simulink model "Robustofinal"  (R2021b)
settings: Solver=VariableStepAuto  StartTime=0.0  StopTime=3  FixedStep=0.000001  RelTol=1e-3
values from neighbouring files (symbols this model uses):
  C = 2500*10^-6    (= 0.0025)    [parametrosRs.m]
  Em = 80    [parametrosRs.m]
  epsilon = 0.1    [parametrosRs.m]
  k1 = 103    [parametrosRs.m]
  k2 = 1000    [parametrosRs.m]
  k3 = 3000    [parametrosRs.m]
  L = 10*10^-3    (= 0.01)    [parametrosRs.m]
  R = 0.1    [parametrosRs.m]
  Rl = 33.33    [parametrosRs.m]
  w = 60    [parametrosRs.m]
  x2d = 0    [parametrosRs.m]
  x3d = 48    [parametrosRs.m]
libraries: spsIGBTDiodeLib x6, eeTransforms x5, spsCurrentMeasurementLib x4, spsSeriesRLCBranchLib x4, spsVoltageMeasurementLib x4, spsACVoltageSourceLib x3, simulink x1, spsDCVoltageSourceLib x1, spsGroundLib x1, spsSVPWMGenerator2LevelLib x1, spsVariableResistorLib x1, spspowerguiLib x1
settings Model: Creator=CIO  LastModifiedBy=LAPONE

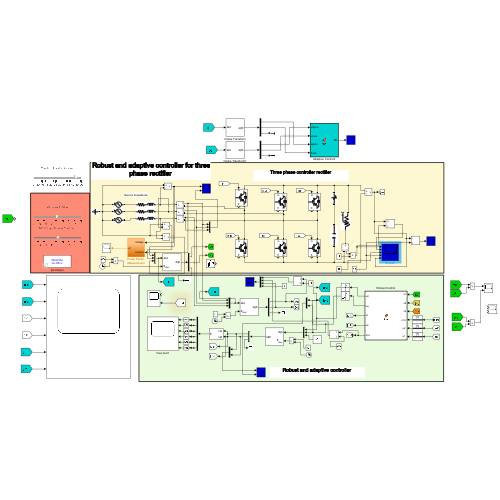
[thumbnail: Simulink's stored preview of the top-level diagram]
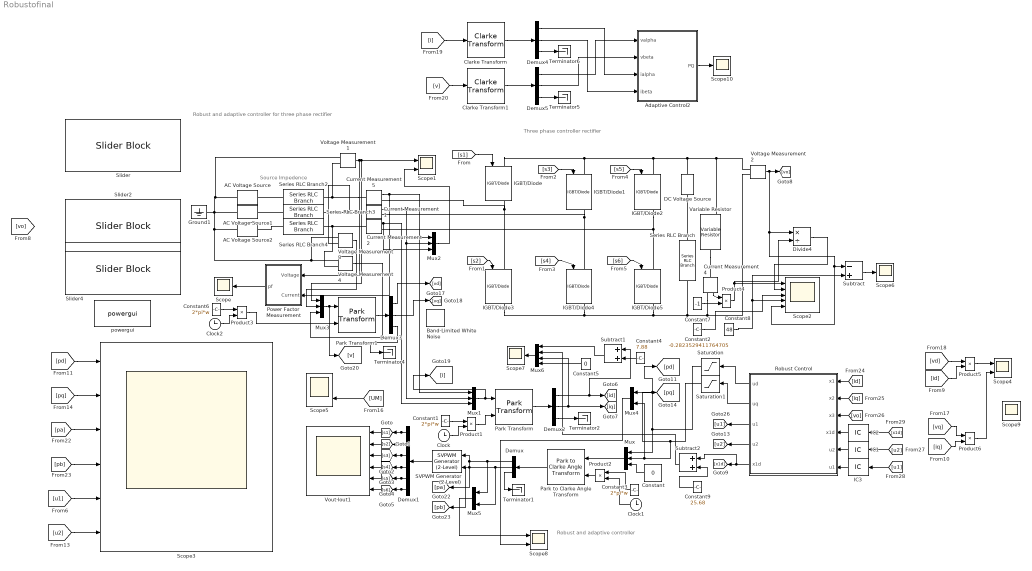
== system Robustofinal ==
  note: Source Impedence
  note: Three phase controller rectifier
  note: Robust and adaptive controller
  note: Robust and adaptive controller for three phase rectifier
  AC Voltage Source : spsACVoltageSourceLib/AC Voltage Source  Amplitude=Em  Phase=0  Frequency=w  SampleTime=0  Measurements=None  BusType=swing  Pref=10e3  Qref=0  Qmin=-inf  Qmax=+inf
  AC Voltage Source1 : spsACVoltageSourceLib/AC Voltage Source  Amplitude=Em  Phase=240  Frequency=w  SampleTime=0  Measurements=None  BusType=swing  Pref=10e3  Qref=0  Qmin=-inf  Qmax=+inf
  AC Voltage Source2 : spsACVoltageSourceLib/AC Voltage Source  Amplitude=Em  Phase=120  Frequency=w  SampleTime=0  Measurements=None  BusType=swing  Pref=10e3  Qref=0  Qmin=-inf  Qmax=+inf
  Adaptive Control2 : MATLAB Function  TreatAsAtomicUnit=on
  Band-Limited White Noise : simulink/Sources/Band-Limited White Noise  Cov=[0.001]  Ts=0.001  seed=[23341]
  Clarke Transform : eeTransforms/Clarke Transform  PowerInvariant=off
      settings: SourceProductBaseCode=PS
  Clarke Transform1 : eeTransforms/Clarke Transform  PowerInvariant=off
      settings: SourceProductBaseCode=PS
  Clock : Clock
  Clock1 : Clock
  Clock2 : Clock
  Constant : Constant  Value=0
  Constant1 : Constant  Value=2*pi*w
  Constant2 : Constant  Value=-0.2823529411764705
  Constant3 : Constant  Value=2*pi*w
  Constant4 : Constant  Value=7.88
  Constant5 : Constant  Value=0
  Constant6 : Constant  Value=2*pi*w
  Constant7 : Constant  Value=-1
  Constant8 : Constant  Value=48
  Constant9 : Constant  Value=25.68
  Current Measurement{1..2,4..5} (4 alike) : spsCurrentMeasurementLib/Current Measurement  PhasorSimulation=off  OutputType=Magnitude  PSBequivalent=0
  DC Voltage Source : spsDCVoltageSourceLib/DC Voltage Source  Amplitude=0.0941176470588232  Measurements=None
  Demux{,2..5} (5 alike) : Demux  Outputs=3
  Demux1 : Demux  Outputs=6
  Divide4 : Product  Inputs=*/
  Ground1 : spsGroundLib/Ground  LConnTagsString=a
  IC1 : InitialCondition
  IC2 : InitialCondition
  IC3 : InitialCondition
  IGBT/Diode{,1..5} (6 alike) : spsIGBTDiodeLib/IGBT//Diode  Ron=1e-3  Rs=1e5  Cs=inf  Measurements=on
  Mux{,1..3} (4 alike) : Mux  Inputs=3
  Mux4 : Mux  Inputs=2
  Mux5 : Mux  Inputs=2
  Mux6 : Mux
  Park Transform : eeTransforms/Park Transform  AxisAlignment=D-axis  PowerInvariant=off
  Park Transform1 : eeTransforms/Park Transform  AxisAlignment=D-axis  PowerInvariant=off
  Park to Clarke Angle Transform : eeTransforms/Park to Clarke Angle Transform  AxisAlignment=D-axis
      settings: SourceProductBaseCode=PS
  Power Factor Measurement : Subsystem
  Product{1..6} (6 alike) : Product
  Robust Control : MATLAB Function  TreatAsAtomicUnit=on
  SVPWM Generator (2-Level) : spsSVPWMGenerator2LevelLib/SVPWM Generator (2-Level)  InputType=alpha-beta components  SwitchingPattern=Pattern #1  Fc=10000  ParUref=[0.8 -30 50]  Ts=0
      settings: SourceProductBaseCode=PS
  Saturation : Saturate  UpperLimit=50  LowerLimit=-50
  Saturation1 : Saturate  UpperLimit=25  LowerLimit=-25
  Scope{,6..7,10} (4 alike) : Scope
  Scope{1,4..5,8..9} (5 alike) : Scope  NumInputPorts=2
  Scope2 : Scope  NumInputPorts=5
  Scope3 : Scope  NumInputPorts=6
  Series RLC Branch : spsSeriesRLCBranchLib/Series RLC Branch  LConnTagsString=__new0  RConnTagsString=__new0  BranchType=C  Resistance=5  Inductance=1e-3  SetiL0=off  InitialCurrent=0  Capacitance=C  Setx0=off  InitialVoltage=0  Measurements=None
  Series RLC Branch2 : spsSeriesRLCBranchLib/Series RLC Branch  LConnTagsString=__new0  RConnTagsString=__new0  BranchType=RL  Resistance=R  Inductance=L  SetiL0=off  InitialCurrent=0  Capacitance=200e-6  Setx0=off  InitialVoltage=0  Measurements=Branch voltage and current
  Series RLC Branch3 : spsSeriesRLCBranchLib/Series RLC Branch  LConnTagsString=__new0  RConnTagsString=__new0  BranchType=RL  Resistance=R  Inductance=L  SetiL0=off  InitialCurrent=0  Capacitance=200e-6  Setx0=off  InitialVoltage=0  Measurements=Branch voltage and current
  Series RLC Branch4 : spsSeriesRLCBranchLib/Series RLC Branch  LConnTagsString=__new0  RConnTagsString=__new0  BranchType=RL  Resistance=R  Inductance=L  SetiL0=off  InitialCurrent=0  Capacitance=200e-6  Setx0=off  InitialVoltage=0  Measurements=Branch voltage and current
  Slider : SliderBlock  ScaleMin=6  ScaleMax=50
  Slider2 : SliderBlock  ScaleMin=-8  ScaleMax=8
  Slider4 : SliderBlock  ScaleMin=-8  ScaleMax=8
  Subtract : Sum  Inputs=-+
  Subtract1 : Sum
  Subtract2 : Sum
  Terminator{1..2,4..6} (5 alike) : Terminator
  Variable Resistor : spsVariableResistorLib/Variable Resistor  Rabsmin=44.92307692307692
      settings: SourceProductBaseCode=PS
  Voltage Measurement{1..4} (4 alike) : spsVoltageMeasurementLib/Voltage Measurement  PhasorSimulation=off  OutputType=Magnitude  PSBequivalent=0
  Vout-Iout1 : Scope  NumInputPorts=6
  powergui : spspowerguiLib/powergui  Priority=1  SimulationMode=Discrete  SampleTime=1e-6  frequency=60  Iterations=50  frequencyindice=0  Pbase=100e6  ErrMax=1e-4  UnitsV=kV  UnitsW=MW  buscounter=0  FunctionMessages=off  echomessages=off  EnableUseOfTLC=off  CurrentSourceSwitches=off  DisableSnubberDevices=off  DisableRonSwitches=off  DisableVfSwitches=off  DisplayEquations=off  AutomaticDiscreteSolvers=off  SolverType=Tustin/Backward Euler (TBE)  Interpol=off  ExternalGateDelay=off  methode=off  Ts=0  x0status=blocks  SPID=off  SwTol=0  HookPort=off  NonlinearTolerance=0  nMaxIteration=15  ContinueOnMaxIteration=off  RestoreLinks=warning  ResistiveCurrentMeasurement=off  Frange=[0:2:500]  Ylog=off  Xlog=on  ShowGrid=off  save=off  variable=ZData  structure=0  ZoomFFT=on  StartTime=0.0  cycles=1  DisplayStyle=1  fundamental=60  FreqAxis=off  MaxFrequency=1000  frequencyindicesteady=1  RmsSteady=1  display=off
  wires:
  Constant4/1 -> Subtract1/2
  Park to Clarke Angle Transform/1 -> Demux/1
  Clock1/1 -> Product2/2
  Product2/1 -> Park to Clarke Angle Transform/2
  Clock/1 -> Product1/2
  Demux2/3 -> Terminator2/1
  Divide4/1 -> Scope2/2
  Product1/1 -> Park Transform/2
  Constant8/1 -> Subtract/2, Scope2/4
  Constant1/1 -> Product1/1
  Current Measurement2/1 -> Mux2/3, Mux1/3
  Constant3/1 -> Product2/1
  [s2] -> IGBT/Diode3/1
  Product4/1 -> Divide4/2, Scope2/1
  Current Measurement5/1 -> Power Factor Measurement/2(Current), Mux2/1, Mux1/1
  Mux4/1 -> Scope8/2
  [s3] -> IGBT/Diode1/1
  Demux1/1 -> Vout-Iout1/1, [s1]
  Mux1/1 -> [i], Park Transform/1
  Demux1/5 -> Vout-Iout1/5, [s5]
  Voltage Measurement1/1 -> Power Factor Measurement/1(Voltage), Scope1/1, Mux3/1
  Current Measurement1/1 -> Mux2/2, Mux1/2
  Constant/1 -> Mux/3
  Saturation/1 -> Mux4/1, [pd], Mux/1
  Subtract/1 -> Scope6/1
  Current Measurement4/1 -> Product4/1
  Mux2/1 -> Scope1/2
  SVPWM Generator (2-Level)/1 -> Demux1/1
  Demux/1 -> Mux5/1, SVPWM Generator (2-Level)/1, [pa]
  [s1] -> IGBT/Diode/1
  Demux2/2 -> Mux6/3, [iq]
  Constant2/1 -> Scope2/3
  [s6] -> IGBT/Diode5/1
  Demux1/2 -> Vout-Iout1/2, [s2]
  [s4] -> IGBT/Diode4/1
  Park Transform/1 -> Demux2/1
  Voltage Measurement2/1 -> Divide4/1, Scope2/5, Subtract/1, [vo]
  Mux/1 -> Park to Clarke Angle Transform/1
  Mux6/1 -> Scope7/1
  Demux1/4 -> Vout-Iout1/4, [s4]
  Demux/2 -> Mux5/2, [pb], SVPWM Generator (2-Level)/2
  Demux1/3 -> Vout-Iout1/3, [s3]
  [s5] -> IGBT/Diode2/1
  Demux1/6 -> Vout-Iout1/6, [s6]
  Saturation1/1 -> [pq], Mux4/2, Mux/2
  Demux/3 -> Terminator1/1
  Mux5/1 -> Scope8/1
  Constant7/1 -> Product4/2
  Power Factor Measurement/1(pf) -> Scope/1
  [UM] -> Scope5/2
  Constant5/1 -> Mux6/4
  Demux2/1 -> Subtract1/1, [id]
  Mux3/1 -> [v], Park Transform1/1
  Park Transform1/1 -> Demux3/1
  Voltage Measurement3/1 -> Mux3/2
  Voltage Measurement4/1 -> Mux3/3
  Clock2/1 -> Product3/2
  Constant6/1 -> Product3/1
  Product3/1 -> Park Transform1/2
  Demux3/3 -> Terminator4/1
  Demux3/1 -> [vd]
  Demux3/2 -> [vq]
  [id] -> Product5/2
  [iq] -> Product6/2
  Product5/1 -> Scope4/1
  Product6/1 -> Scope4/2
  [vd] -> Product5/1
  [vq] -> Product6/1
  Clarke Transform/1 -> Demux4/1
  Clarke Transform1/1 -> Demux5/1
  Demux5/3 -> Terminator5/1
  Demux4/3 -> Terminator6/1
  [i] -> Clarke Transform/1
  [v] -> Clarke Transform1/1
  Demux4/1 -> Adaptive Control2/3(ialpha)
  Demux4/2 -> Adaptive Control2/4(ibeta)
  Demux5/1 -> Adaptive Control2/1(valpha)
  Demux5/2 -> Adaptive Control2/2(vbeta)
  Adaptive Control2/1(PQ) -> Scope10/1
  [x1d] -> IC2/1
  IC2/1 -> Robust Control/4("x1d ")
  [u2] -> IC1/1
  IC1/1 -> Robust Control/5("u2 ")
  [vo] -> Robust Control/3(x3)
  [id] -> Robust Control/1(x1)
  IC3/1 -> Robust Control/6("u1 ")
  [u1] -> IC3/1
  [iq] -> Robust Control/2(x2)
  Robust Control/3(u1) -> [u1]
  Robust Control/4(u2) -> [u2]
  Robust Control/1(ud) -> Saturation/1
  Robust Control/2(uq) -> Saturation1/1
  [pd] -> Scope3/1
  [pq] -> Scope3/2
  [pb] -> Scope3/4
  [pa] -> Scope3/3
  [u2] -> Scope3/6
  [u1] -> Scope3/5
  Subtract1/1 -> Mux6/1
  Constant9/1 -> Subtract2/2
  Robust Control/5(x1d) -> Subtract2/1, [x1d]
  Subtract2/1 -> Mux6/2
  connections:
  IGBT/Diode/RConn1 -- IGBT/Diode3/LConn1 -- Current Measurement5/RConn1
  Current Measurement5/LConn1 -- Series RLC Branch2/RConn1 -- Voltage Measurement1/LConn2
  Current Measurement4/RConn1 -- IGBT/Diode4/RConn1 -- IGBT/Diode3/RConn1 -- IGBT/Diode5/RConn1 -- Series RLC Branch/RConn1 -- Voltage Measurement2/LConn2
  Current Measurement2/RConn1 -- IGBT/Diode2/RConn1 -- IGBT/Diode5/LConn1
  Current Measurement1/RConn1 -- IGBT/Diode1/RConn1 -- IGBT/Diode4/LConn1
  AC Voltage Source1/RConn1 -- Voltage Measurement3/LConn1 -- Voltage Measurement4/LConn1 -- AC Voltage Source2/RConn1 -- Ground1/LConn1 -- Voltage Measurement1/LConn1 -- AC Voltage Source/RConn1
  Voltage Measurement2/LConn1 -- Variable Resistor/LConn1 -- DC Voltage Source/RConn1 -- IGBT/Diode2/LConn1 -- IGBT/Diode/LConn1 -- IGBT/Diode1/LConn1
  Series RLC Branch3/LConn1 -- AC Voltage Source1/LConn1
  Variable Resistor/RConn1 -- Current Measurement4/LConn1
  Series RLC Branch4/RConn1 -- Voltage Measurement4/LConn2 -- Current Measurement2/LConn1
  Series RLC Branch3/RConn1 -- Voltage Measurement3/LConn2 -- Current Measurement1/LConn1
  Series RLC Branch2/LConn1 -- AC Voltage Source/LConn1
  Series RLC Branch4/LConn1 -- AC Voltage Source2/LConn1
  Series RLC Branch/LConn1 -- DC Voltage Source/LConn1

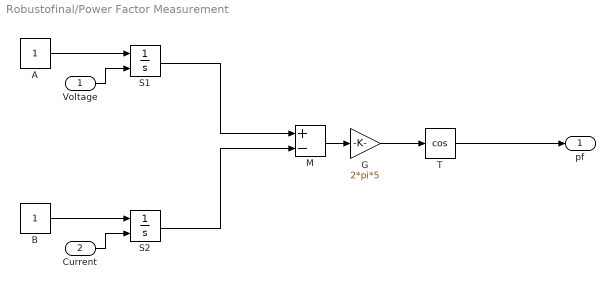
== system Robustofinal/Power Factor Measurement ==
  Voltage : Inport
  Current : Inport  Port=2
  A : Constant
  B : Constant
  G : Gain  Gain=2*pi*5
  M : Sum  Inputs=+-
  S1 : Integrator  ExternalReset=falling
  S2 : Integrator  ExternalReset=falling
  T : Trigonometry  Operator=cos
  pf : Outport
  wires:
  A/1 -> S1/1
  B/1 -> S2/1
  S1/1 -> M/1
  S2/1 -> M/2
  Voltage/1 -> S1/2
  Current/1 -> S2/2
  M/1 -> G/1
  G/1 -> T/1
  T/1 -> pf/1

== matlab function Robustofinal/Adaptive Control2 ==
  data: valpha input; PQ output; vbeta input; ialpha input; ibeta input
function PQ  = fcn(valpha,vbeta,ialpha,ibeta)


PQ = [valpha,vbeta;vbeta,-valpha]*[ialpha;ibeta];

== matlab function Robustofinal/Robust Control ==
  data: x1 input; ud output; x2 input; x3 input; uq output; Em parameter; C parameter; L parameter; w parameter; R parameter; x3d parameter; x2d parameter; k3 parameter; k2 parameter; Rl parameter; u1 output; u2 output; x1d input; k1 parameter; x1d output; u2 input; u1 input; epsilon parameter
function [ud , uq, u1,u2,x1d] = fcn(x1, x2, x3,Em,C, L, w, R, x3d, x2d,k3, k2,Rl,x1d, k1,u2,u1,epsilon)

e1 = x1 - x1d; e2 = x2 - x2d;      e3 = x3 - x3d; 


%x1d = ((1/2*L)/(3/(4*C)))*(u2/u1)*(x3);
%x1d = (u2/u1)+( Em/(2*R)) - (sqrt((Em)^2 - (8*R*x3d^2)/(3*Rl)))/(2*R);
%x1d = (2*C*u2*(e3 + x3d))/(3*L*u1) - e1;
x1d = Em/(2*R) - (sqrt((Em)^2 - (8*R*x3d^2)/(3*Rl)))/(2*R);


%controls
%para evitar singularidades agregamos el termino epsilon donde corresponda


%uq = (2*L/(x3 + epsilon)) * ( -(R/L)*(e2 + x2d) + w*(e1 + x1d) + k2*sqrt(abs(e2))*sign(e2) );
 uq = (2*L/(x3 + epsilon)) * ( -(R/L)*(e2) + w*(e1 + x1d) + k2*sqrt(abs(e2))*sign(e2) );


u1 = ((-R/L)*(e1+x1d)) - (w*e2) + (Em/L) + (k1*sqrt(abs(e1))*sign(e1));
%u1 = ((-R/L)*(e1+x1d)) + (Em/L) + (k1*sqrt(abs(e1))*sign(e1));

%u2 = -(3/(4*C))*(e2 + x2d)*uq + (1/(Rl*C)) * (e3 + x3d) - k3*sqrt(abs(e3))*sign(e3);
%u2 = +(1/(Rl*C)) * (e3 + x3d) - k3*sqrt(abs(e3))*sign(e3);
u2 = -(3/(4*C))*(e2)*uq + (1/(Rl*C)) * (e3 + x3d) - k3*sqrt(abs(e3))*sign(e3);

ud =  ((4*C)/3) * u2/(x1 + epsilon) ;
 %ud =  ((2*L)/1) * u1/(e3 + x3d + epsilon) ;
